simulink model "lab4_quaternions"  (R2021b)
settings: Solver=VariableStepAuto  StartTime=0.0  StopTime=10.0  RelTol=1e-3
values from neighbouring files (symbols this model uses):
  J = [Ixx 0 0; 0 Iyy 0; 0 0 Izz]    [lab4_task1and2.m]    (also in lab4_task3.m)
  Jinv = inv(J)    [lab4_task1and2.m]    (also in lab4_task3.m)
  q0 = [e(1)*sin(phi/2); e(2)*sin(phi/2); e(3)*sin(phi/2); cos(phi/2)]    [lab4_task3.m]
  w0 = [0.45 0.52 0.55]'    [lab4_task1and2.m]    (also in lab4_task3.m)
libraries: matrix_library x1
settings Model: Creator=samuz  LastModifiedBy=samuz

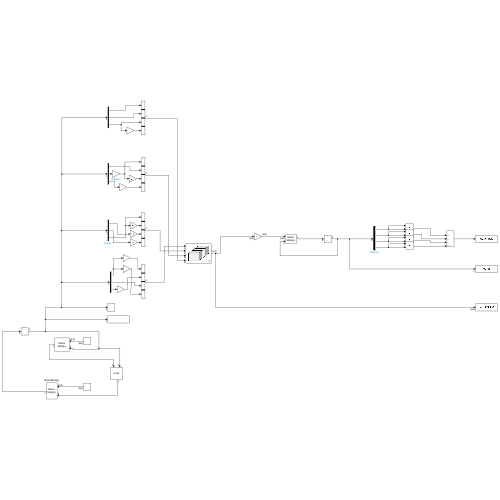
[thumbnail: Simulink's stored preview of the top-level diagram]
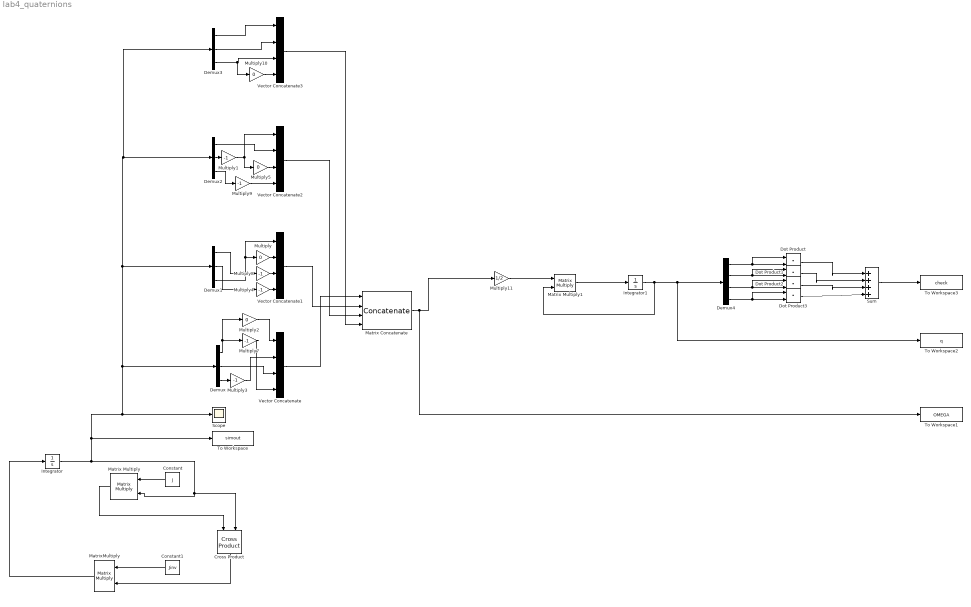
== system lab4_quaternions ==
  Constant : Constant  Value=J
  Constant1 : Constant  Value=Jinv
  Cross Product : matrix_library/Cross Product
      settings: SourceProductBaseCode=SL
  Demux{,1..3} (4 alike) : Demux  Outputs=3
  Demux4 : Demux
  Dot Product{,1..3} (4 alike) : DotProduct  InputSameDT=on  OutDataTypeStr=Inherit: Inherit via internal rule
  Integrator : Integrator  InitialCondition=w0
  Integrator1 : Integrator  InitialCondition=q0
  Matrix Concatenate : Concatenate  NumInputs=4  Mode=Multidimensional array  ConcatenateDimension=2
  Matrix Multiply : Product  Multiplication=Matrix(*)
  Matrix Multiply1 : Product  Multiplication=Matrix(*)
  MatrixMultiply : Product  Multiplication=Matrix(*)
  Multiply{,2,5,10} (4 alike) : Gain  Gain=0
  Multiply{1,3..4,7..9} (6 alike) : Gain  Gain=-1
  Multiply11 : Gain  Gain=1/2
  Scope : Scope
  Sum : Sum  Inputs=|++++
  To Workspace : ToWorkspace  VariableName=simout  SampleTime=-1
  To Workspace1 : ToWorkspace  VariableName=OMEGA  SampleTime=-1
  To Workspace2 : ToWorkspace  VariableName=q  SampleTime=-1
  To Workspace3 : ToWorkspace  VariableName=check  SampleTime=-1
  Vector Concatenate{,1..3} (4 alike) : Concatenate  NumInputs=4
  wires:
  Constant/1 -> Matrix Multiply/1
  MatrixMultiply/1 -> Integrator/1
  Constant1/1 -> MatrixMultiply/1
  Cross Product/1 -> MatrixMultiply/2
  Matrix Multiply/1 -> Cross Product/1
  Integrator/1 -> To Workspace/1, Demux3/1, Demux2/1, Demux1/1, Demux/1, Scope/1, Cross Product/2, Matrix Multiply/2
  Vector Concatenate1/1 -> Matrix Concatenate/2
  Vector Concatenate/1 -> Matrix Concatenate/1
  Demux/1 -> Multiply2/1, Multiply7/1
  Multiply2/1 -> Vector Concatenate/1
  Vector Concatenate2/1 -> Matrix Concatenate/3
  Matrix Concatenate/1 -> Multiply11/1, To Workspace1/1
  Matrix Multiply1/1 -> Integrator1/1
  Integrator1/1 -> Matrix Multiply1/2, Demux4/1, To Workspace2/1
  Demux/3 -> Multiply3/1
  Multiply3/1 -> Vector Concatenate/2
  Demux/2 -> Vector Concatenate/3
  Multiply7/1 -> Vector Concatenate/4
  Demux1/3 -> Multiply/1, Vector Concatenate1/1
  Multiply/1 -> Vector Concatenate1/2
  Multiply4/1 -> Vector Concatenate1/4
  Multiply8/1 -> Vector Concatenate1/3
  Demux1/1 -> Multiply8/1
  Demux1/2 -> Multiply4/1
  Demux2/2 -> Multiply1/1
  Multiply1/1 -> Multiply5/1, Vector Concatenate2/1
  Demux2/1 -> Vector Concatenate2/2
  Multiply5/1 -> Vector Concatenate2/3
  Demux2/3 -> Multiply9/1
  Multiply9/1 -> Vector Concatenate2/4
  Demux3/1 -> Vector Concatenate3/1
  Demux3/2 -> Vector Concatenate3/2
  Demux3/3 -> Multiply10/1, Vector Concatenate3/3
  Multiply10/1 -> Vector Concatenate3/4
  Vector Concatenate3/1 -> Matrix Concatenate/4
  Multiply11/1 -> Matrix Multiply1/1
  Demux4/1 -> Dot Product/1, Dot Product/2
  Demux4/2 -> Dot Product1/1, Dot Product1/2
  Demux4/3 -> Dot Product2/1, Dot Product2/2
  Demux4/4 -> Dot Product3/1, Dot Product3/2
  Dot Product/1 -> Sum/1
  Dot Product1/1 -> Sum/2
  Dot Product2/1 -> Sum/3
  Dot Product3/1 -> Sum/4
  Sum/1 -> To Workspace3/1
